simulink model "rx2"  (R2022b)
settings: Solver=FixedStepDiscrete  StartTime=0.0  StopTime=3.3E6  FixedStep=1  RelTol=1e-3  EnableMultiTasking=on
model workspace (MAT data in the model file):
  mwTaskManagerKernelLatency = 0
undefined symbols (not defined in the file or in its folder): Add, jsin, magnitude, rom_pilot_conj_tt, Shift
libraries: hdlsllib x3231, whdlutilities x525, simulink x260, whdlmod x112, whdledac x26, dsphdlmathfun2 x24, commchan3 x1
(part 17 of 59)

== system rx2/process divide/transport_block1/Subsystem2/ctrl_gen ==
  data_in : Inport
  valid_in : Inport  Port=2
  Delay : Delay  DelayLength=1  InitialCondition=0
  Delay1 : Delay  DelayLength=1  InitialCondition=0
  Delay2 : Delay  DelayLength=1  InitialCondition=0
  Detect Fall Nonpositive : hdlsllib/Logic and Bit Operations/Detect Fall Nonpositive  vinit=0  OutDataTypeStr=boolean
  Detect Rise Positive : hdlsllib/Logic and Bit Operations/Detect Rise Positive  vinit=0  OutDataTypeStr=boolean
  Sample Control Bus Creator : whdlutilities/Sample Control Bus Creator
  data_out : Outport
  ctrl_out : Outport  Port=2
  wires:
  Detect Rise Positive/1 -> Sample Control Bus Creator/1
  Delay2/1 -> data_out/1
  data_in/1 -> Delay2/1
  Delay1/1 -> Detect Rise Positive/1
  Delay/1 -> Sample Control Bus Creator/3
  Sample Control Bus Creator/1 -> ctrl_out/1
  valid_in/1 -> Delay1/1, Detect Fall Nonpositive/1, Delay/1
  Detect Fall Nonpositive/1 -> Sample Control Bus Creator/2

== system rx2/process divide/transport_block1/Subsystem3/ctrl_gen ==
  data_in : Inport
  valid_in : Inport  Port=2
  Delay : Delay  DelayLength=1  InitialCondition=0
  Delay1 : Delay  DelayLength=1  InitialCondition=0
  Delay2 : Delay  DelayLength=1  InitialCondition=0
  Detect Fall Nonpositive : hdlsllib/Logic and Bit Operations/Detect Fall Nonpositive  vinit=0  OutDataTypeStr=boolean
  Detect Rise Positive : hdlsllib/Logic and Bit Operations/Detect Rise Positive  vinit=0  OutDataTypeStr=boolean
  Sample Control Bus Creator : whdlutilities/Sample Control Bus Creator
  data_out : Outport
  ctrl_out : Outport  Port=2
  wires:
  Detect Fall Nonpositive/1 -> Sample Control Bus Creator/2
  valid_in/1 -> Delay/1, Detect Fall Nonpositive/1, Delay1/1
  Sample Control Bus Creator/1 -> ctrl_out/1
  Delay/1 -> Sample Control Bus Creator/3
  Delay1/1 -> Detect Rise Positive/1
  data_in/1 -> Delay2/1
  Delay2/1 -> data_out/1
  Detect Rise Positive/1 -> Sample Control Bus Creator/1

== system rx2/process divide/transport_block1/Subsystem4/ctrl_gen ==
  data_in : Inport
  valid_in : Inport  Port=2
  Delay : Delay  DelayLength=1  InitialCondition=0
  Delay1 : Delay  DelayLength=1  InitialCondition=0
  Delay2 : Delay  DelayLength=1  InitialCondition=0
  Detect Fall Nonpositive : hdlsllib/Logic and Bit Operations/Detect Fall Nonpositive  vinit=0  OutDataTypeStr=boolean
  Detect Rise Positive : hdlsllib/Logic and Bit Operations/Detect Rise Positive  vinit=0  OutDataTypeStr=boolean
  Sample Control Bus Creator : whdlutilities/Sample Control Bus Creator
  data_out : Outport
  ctrl_out : Outport  Port=2
  wires:
  Detect Rise Positive/1 -> Sample Control Bus Creator/1
  Delay2/1 -> data_out/1
  data_in/1 -> Delay2/1
  Delay1/1 -> Detect Rise Positive/1
  Delay/1 -> Sample Control Bus Creator/3
  Sample Control Bus Creator/1 -> ctrl_out/1
  valid_in/1 -> Delay1/1, Detect Fall Nonpositive/1, Delay/1
  Detect Fall Nonpositive/1 -> Sample Control Bus Creator/2

== system rx2/process divide/transport_block1/Subsystem5/ctrl_gen ==
  data_in : Inport
  valid_in : Inport  Port=2
  Delay : Delay  DelayLength=1  InitialCondition=0
  Delay1 : Delay  DelayLength=1  InitialCondition=0
  Delay2 : Delay  DelayLength=1  InitialCondition=0
  Detect Fall Nonpositive : hdlsllib/Logic and Bit Operations/Detect Fall Nonpositive  vinit=0  OutDataTypeStr=boolean
  Detect Rise Positive : hdlsllib/Logic and Bit Operations/Detect Rise Positive  vinit=0  OutDataTypeStr=boolean
  Sample Control Bus Creator : whdlutilities/Sample Control Bus Creator
  data_out : Outport
  ctrl_out : Outport  Port=2
  wires:
  Detect Rise Positive/1 -> Sample Control Bus Creator/1
  Delay2/1 -> data_out/1
  data_in/1 -> Delay2/1
  Delay1/1 -> Detect Rise Positive/1
  Delay/1 -> Sample Control Bus Creator/3
  Sample Control Bus Creator/1 -> ctrl_out/1
  valid_in/1 -> Delay1/1, Detect Fall Nonpositive/1, Delay/1
  Detect Fall Nonpositive/1 -> Sample Control Bus Creator/2

== system rx2/process divide/transport_block1/Subsystem6/ctrl_gen ==
  data_in : Inport
  valid_in : Inport  Port=2
  Delay : Delay  DelayLength=1  InitialCondition=0
  Delay1 : Delay  DelayLength=1  InitialCondition=0
  Delay2 : Delay  DelayLength=1  InitialCondition=0
  Detect Fall Nonpositive : hdlsllib/Logic and Bit Operations/Detect Fall Nonpositive  vinit=0  OutDataTypeStr=boolean
  Detect Rise Positive : hdlsllib/Logic and Bit Operations/Detect Rise Positive  vinit=0  OutDataTypeStr=boolean
  Sample Control Bus Creator : whdlutilities/Sample Control Bus Creator
  data_out : Outport
  ctrl_out : Outport  Port=2
  wires:
  Detect Rise Positive/1 -> Sample Control Bus Creator/1
  Delay2/1 -> data_out/1
  data_in/1 -> Delay2/1
  Delay1/1 -> Detect Rise Positive/1
  Delay/1 -> Sample Control Bus Creator/3
  Sample Control Bus Creator/1 -> ctrl_out/1
  valid_in/1 -> Delay1/1, Detect Fall Nonpositive/1, Delay/1
  Detect Fall Nonpositive/1 -> Sample Control Bus Creator/2

== system rx2/process divide/transport_block1/Subsystem7/ctrl_gen ==
  data_in : Inport
  valid_in : Inport  Port=2
  Delay : Delay  DelayLength=1  InitialCondition=0
  Delay1 : Delay  DelayLength=1  InitialCondition=0
  Delay2 : Delay  DelayLength=1  InitialCondition=0
  Detect Fall Nonpositive : hdlsllib/Logic and Bit Operations/Detect Fall Nonpositive  vinit=0  OutDataTypeStr=boolean
  Detect Rise Positive : hdlsllib/Logic and Bit Operations/Detect Rise Positive  vinit=0  OutDataTypeStr=boolean
  Sample Control Bus Creator : whdlutilities/Sample Control Bus Creator
  data_out : Outport
  ctrl_out : Outport  Port=2
  wires:
  Detect Rise Positive/1 -> Sample Control Bus Creator/1
  Delay2/1 -> data_out/1
  data_in/1 -> Delay2/1
  Delay1/1 -> Detect Rise Positive/1
  Delay/1 -> Sample Control Bus Creator/3
  Sample Control Bus Creator/1 -> ctrl_out/1
  valid_in/1 -> Delay1/1, Detect Fall Nonpositive/1, Delay/1
  Detect Fall Nonpositive/1 -> Sample Control Bus Creator/2

== system rx2/process divide/transport_block1/Subsystem8/ctrl_gen ==
  data_in : Inport
  valid_in : Inport  Port=2
  Delay : Delay  DelayLength=1  InitialCondition=0
  Delay1 : Delay  DelayLength=1  InitialCondition=0
  Delay2 : Delay  DelayLength=1  InitialCondition=0
  Detect Fall Nonpositive : hdlsllib/Logic and Bit Operations/Detect Fall Nonpositive  vinit=0  OutDataTypeStr=boolean
  Detect Rise Positive : hdlsllib/Logic and Bit Operations/Detect Rise Positive  vinit=0  OutDataTypeStr=boolean
  Sample Control Bus Creator : whdlutilities/Sample Control Bus Creator
  data_out : Outport
  ctrl_out : Outport  Port=2
  wires:
  Detect Rise Positive/1 -> Sample Control Bus Creator/1
  Delay2/1 -> data_out/1
  data_in/1 -> Delay2/1
  Delay1/1 -> Detect Rise Positive/1
  Delay/1 -> Sample Control Bus Creator/3
  Sample Control Bus Creator/1 -> ctrl_out/1
  valid_in/1 -> Delay1/1, Detect Fall Nonpositive/1, Delay/1
  Detect Fall Nonpositive/1 -> Sample Control Bus Creator/2

== system rx2/process divide/transport_block1/Subsystem9/ctrl_gen ==
  data_in : Inport
  valid_in : Inport  Port=2
  Delay : Delay  DelayLength=1  InitialCondition=0
  Delay1 : Delay  DelayLength=1  InitialCondition=0
  Delay2 : Delay  DelayLength=1  InitialCondition=0
  Detect Fall Nonpositive : hdlsllib/Logic and Bit Operations/Detect Fall Nonpositive  vinit=0  OutDataTypeStr=boolean
  Detect Rise Positive : hdlsllib/Logic and Bit Operations/Detect Rise Positive  vinit=0  OutDataTypeStr=boolean
  Sample Control Bus Creator : whdlutilities/Sample Control Bus Creator
  data_out : Outport
  ctrl_out : Outport  Port=2
  wires:
  Detect Rise Positive/1 -> Sample Control Bus Creator/1
  Delay2/1 -> data_out/1
  data_in/1 -> Delay2/1
  Delay1/1 -> Detect Rise Positive/1
  Delay/1 -> Sample Control Bus Creator/3
  Sample Control Bus Creator/1 -> ctrl_out/1
  valid_in/1 -> Delay1/1, Detect Fall Nonpositive/1, Delay/1
  Detect Fall Nonpositive/1 -> Sample Control Bus Creator/2

== system rx2/process divide/transport_block2/Subsystem1/ctrl_gen ==
  data_in : Inport
  valid_in : Inport  Port=2
  Delay : Delay  DelayLength=1  InitialCondition=0
  Delay1 : Delay  DelayLength=1  InitialCondition=0
  Delay2 : Delay  DelayLength=1  InitialCondition=0
  Detect Fall Nonpositive : hdlsllib/Logic and Bit Operations/Detect Fall Nonpositive  vinit=0  OutDataTypeStr=boolean
  Detect Rise Positive : hdlsllib/Logic and Bit Operations/Detect Rise Positive  vinit=0  OutDataTypeStr=boolean
  Sample Control Bus Creator : whdlutilities/Sample Control Bus Creator
  data_out : Outport
  ctrl_out : Outport  Port=2
  wires:
  Detect Rise Positive/1 -> Sample Control Bus Creator/1
  Delay2/1 -> data_out/1
  data_in/1 -> Delay2/1
  Delay1/1 -> Detect Rise Positive/1
  Delay/1 -> Sample Control Bus Creator/3
  Sample Control Bus Creator/1 -> ctrl_out/1
  valid_in/1 -> Delay1/1, Detect Fall Nonpositive/1, Delay/1
  Detect Fall Nonpositive/1 -> Sample Control Bus Creator/2

== system rx2/process divide/transport_block2/Subsystem10/ctrl_gen ==
  data_in : Inport
  valid_in : Inport  Port=2
  Delay : Delay  DelayLength=1  InitialCondition=0
  Delay1 : Delay  DelayLength=1  InitialCondition=0
  Delay2 : Delay  DelayLength=1  InitialCondition=0
  Detect Fall Nonpositive : hdlsllib/Logic and Bit Operations/Detect Fall Nonpositive  vinit=0  OutDataTypeStr=boolean
  Detect Rise Positive : hdlsllib/Logic and Bit Operations/Detect Rise Positive  vinit=0  OutDataTypeStr=boolean
  Sample Control Bus Creator : whdlutilities/Sample Control Bus Creator
  data_out : Outport
  ctrl_out : Outport  Port=2
  wires:
  Detect Fall Nonpositive/1 -> Sample Control Bus Creator/2
  valid_in/1 -> Delay/1, Detect Fall Nonpositive/1, Delay1/1
  Sample Control Bus Creator/1 -> ctrl_out/1
  Delay/1 -> Sample Control Bus Creator/3
  Delay1/1 -> Detect Rise Positive/1
  data_in/1 -> Delay2/1
  Delay2/1 -> data_out/1
  Detect Rise Positive/1 -> Sample Control Bus Creator/1

== system rx2/process divide/transport_block2/Subsystem11/ctrl_gen ==
  data_in : Inport
  valid_in : Inport  Port=2
  Delay : Delay  DelayLength=1  InitialCondition=0
  Delay1 : Delay  DelayLength=1  InitialCondition=0
  Delay2 : Delay  DelayLength=1  InitialCondition=0
  Detect Fall Nonpositive : hdlsllib/Logic and Bit Operations/Detect Fall Nonpositive  vinit=0  OutDataTypeStr=boolean
  Detect Rise Positive : hdlsllib/Logic and Bit Operations/Detect Rise Positive  vinit=0  OutDataTypeStr=boolean
  Sample Control Bus Creator : whdlutilities/Sample Control Bus Creator
  data_out : Outport
  ctrl_out : Outport  Port=2
  wires:
  Detect Fall Nonpositive/1 -> Sample Control Bus Creator/2
  valid_in/1 -> Delay/1, Detect Fall Nonpositive/1, Delay1/1
  Sample Control Bus Creator/1 -> ctrl_out/1
  Delay/1 -> Sample Control Bus Creator/3
  Delay1/1 -> Detect Rise Positive/1
  data_in/1 -> Delay2/1
  Delay2/1 -> data_out/1
  Detect Rise Positive/1 -> Sample Control Bus Creator/1

== system rx2/process divide/transport_block2/Subsystem12/ctrl_gen ==
  data_in : Inport
  valid_in : Inport  Port=2
  Delay : Delay  DelayLength=1  InitialCondition=0
  Delay1 : Delay  DelayLength=1  InitialCondition=0
  Delay2 : Delay  DelayLength=1  InitialCondition=0
  Detect Fall Nonpositive : hdlsllib/Logic and Bit Operations/Detect Fall Nonpositive  vinit=0  OutDataTypeStr=boolean
  Detect Rise Positive : hdlsllib/Logic and Bit Operations/Detect Rise Positive  vinit=0  OutDataTypeStr=boolean
  Sample Control Bus Creator : whdlutilities/Sample Control Bus Creator
  data_out : Outport
  ctrl_out : Outport  Port=2
  wires:
  Detect Fall Nonpositive/1 -> Sample Control Bus Creator/2
  valid_in/1 -> Delay/1, Detect Fall Nonpositive/1, Delay1/1
  Sample Control Bus Creator/1 -> ctrl_out/1
  Delay/1 -> Sample Control Bus Creator/3
  Delay1/1 -> Detect Rise Positive/1
  data_in/1 -> Delay2/1
  Delay2/1 -> data_out/1
  Detect Rise Positive/1 -> Sample Control Bus Creator/1

== system rx2/process divide/transport_block2/Subsystem13/ctrl_gen ==
  data_in : Inport
  valid_in : Inport  Port=2
  Delay : Delay  DelayLength=1  InitialCondition=0
  Delay1 : Delay  DelayLength=1  InitialCondition=0
  Delay2 : Delay  DelayLength=1  InitialCondition=0
  Detect Fall Nonpositive : hdlsllib/Logic and Bit Operations/Detect Fall Nonpositive  vinit=0  OutDataTypeStr=boolean
  Detect Rise Positive : hdlsllib/Logic and Bit Operations/Detect Rise Positive  vinit=0  OutDataTypeStr=boolean
  Sample Control Bus Creator : whdlutilities/Sample Control Bus Creator
  data_out : Outport
  ctrl_out : Outport  Port=2
  wires:
  Detect Fall Nonpositive/1 -> Sample Control Bus Creator/2
  valid_in/1 -> Delay/1, Detect Fall Nonpositive/1, Delay1/1
  Sample Control Bus Creator/1 -> ctrl_out/1
  Delay/1 -> Sample Control Bus Creator/3
  Delay1/1 -> Detect Rise Positive/1
  data_in/1 -> Delay2/1
  Delay2/1 -> data_out/1
  Detect Rise Positive/1 -> Sample Control Bus Creator/1

== system rx2/process divide/transport_block2/Subsystem14/ctrl_gen ==
  data_in : Inport
  valid_in : Inport  Port=2
  Delay : Delay  DelayLength=1  InitialCondition=0
  Delay1 : Delay  DelayLength=1  InitialCondition=0
  Delay2 : Delay  DelayLength=1  InitialCondition=0
  Detect Fall Nonpositive : hdlsllib/Logic and Bit Operations/Detect Fall Nonpositive  vinit=0  OutDataTypeStr=boolean
  Detect Rise Positive : hdlsllib/Logic and Bit Operations/Detect Rise Positive  vinit=0  OutDataTypeStr=boolean
  Sample Control Bus Creator : whdlutilities/Sample Control Bus Creator
  data_out : Outport
  ctrl_out : Outport  Port=2
  wires:
  Detect Fall Nonpositive/1 -> Sample Control Bus Creator/2
  valid_in/1 -> Delay/1, Detect Fall Nonpositive/1, Delay1/1
  Sample Control Bus Creator/1 -> ctrl_out/1
  Delay/1 -> Sample Control Bus Creator/3
  Delay1/1 -> Detect Rise Positive/1
  data_in/1 -> Delay2/1
  Delay2/1 -> data_out/1
  Detect Rise Positive/1 -> Sample Control Bus Creator/1

== system rx2/process divide/transport_block2/Subsystem2/ctrl_gen ==
  data_in : Inport
  valid_in : Inport  Port=2
  Delay : Delay  DelayLength=1  InitialCondition=0
  Delay1 : Delay  DelayLength=1  InitialCondition=0
  Delay2 : Delay  DelayLength=1  InitialCondition=0
  Detect Fall Nonpositive : hdlsllib/Logic and Bit Operations/Detect Fall Nonpositive  vinit=0  OutDataTypeStr=boolean
  Detect Rise Positive : hdlsllib/Logic and Bit Operations/Detect Rise Positive  vinit=0  OutDataTypeStr=boolean
  Sample Control Bus Creator : whdlutilities/Sample Control Bus Creator
  data_out : Outport
  ctrl_out : Outport  Port=2
  wires:
  Detect Fall Nonpositive/1 -> Sample Control Bus Creator/2
  valid_in/1 -> Delay/1, Detect Fall Nonpositive/1, Delay1/1
  Sample Control Bus Creator/1 -> ctrl_out/1
  Delay/1 -> Sample Control Bus Creator/3
  Delay1/1 -> Detect Rise Positive/1
  data_in/1 -> Delay2/1
  Delay2/1 -> data_out/1
  Detect Rise Positive/1 -> Sample Control Bus Creator/1

== system rx2/process divide/transport_block2/Subsystem3/ctrl_gen ==
  data_in : Inport
  valid_in : Inport  Port=2
  Delay : Delay  DelayLength=1  InitialCondition=0
  Delay1 : Delay  DelayLength=1  InitialCondition=0
  Delay2 : Delay  DelayLength=1  InitialCondition=0
  Detect Fall Nonpositive : hdlsllib/Logic and Bit Operations/Detect Fall Nonpositive  vinit=0  OutDataTypeStr=boolean
  Detect Rise Positive : hdlsllib/Logic and Bit Operations/Detect Rise Positive  vinit=0  OutDataTypeStr=boolean
  Sample Control Bus Creator : whdlutilities/Sample Control Bus Creator
  data_out : Outport
  ctrl_out : Outport  Port=2
  wires:
  Detect Rise Positive/1 -> Sample Control Bus Creator/1
  Delay2/1 -> data_out/1
  data_in/1 -> Delay2/1
  Delay1/1 -> Detect Rise Positive/1
  Delay/1 -> Sample Control Bus Creator/3
  Sample Control Bus Creator/1 -> ctrl_out/1
  valid_in/1 -> Delay1/1, Detect Fall Nonpositive/1, Delay/1
  Detect Fall Nonpositive/1 -> Sample Control Bus Creator/2

== system rx2/process divide/transport_block2/Subsystem4/ctrl_gen ==
  data_in : Inport
  valid_in : Inport  Port=2
  Delay : Delay  DelayLength=1  InitialCondition=0
  Delay1 : Delay  DelayLength=1  InitialCondition=0
  Delay2 : Delay  DelayLength=1  InitialCondition=0
  Detect Fall Nonpositive : hdlsllib/Logic and Bit Operations/Detect Fall Nonpositive  vinit=0  OutDataTypeStr=boolean
  Detect Rise Positive : hdlsllib/Logic and Bit Operations/Detect Rise Positive  vinit=0  OutDataTypeStr=boolean
  Sample Control Bus Creator : whdlutilities/Sample Control Bus Creator
  data_out : Outport
  ctrl_out : Outport  Port=2
  wires:
  Detect Fall Nonpositive/1 -> Sample Control Bus Creator/2
  valid_in/1 -> Delay/1, Detect Fall Nonpositive/1, Delay1/1
  Sample Control Bus Creator/1 -> ctrl_out/1
  Delay/1 -> Sample Control Bus Creator/3
  Delay1/1 -> Detect Rise Positive/1
  data_in/1 -> Delay2/1
  Delay2/1 -> data_out/1
  Detect Rise Positive/1 -> Sample Control Bus Creator/1

== system rx2/process divide/transport_block2/Subsystem5/ctrl_gen ==
  data_in : Inport
  valid_in : Inport  Port=2
  Delay : Delay  DelayLength=1  InitialCondition=0
  Delay1 : Delay  DelayLength=1  InitialCondition=0
  Delay2 : Delay  DelayLength=1  InitialCondition=0
  Detect Fall Nonpositive : hdlsllib/Logic and Bit Operations/Detect Fall Nonpositive  vinit=0  OutDataTypeStr=boolean
  Detect Rise Positive : hdlsllib/Logic and Bit Operations/Detect Rise Positive  vinit=0  OutDataTypeStr=boolean
  Sample Control Bus Creator : whdlutilities/Sample Control Bus Creator
  data_out : Outport
  ctrl_out : Outport  Port=2
  wires:
  Detect Fall Nonpositive/1 -> Sample Control Bus Creator/2
  valid_in/1 -> Delay/1, Detect Fall Nonpositive/1, Delay1/1
  Sample Control Bus Creator/1 -> ctrl_out/1
  Delay/1 -> Sample Control Bus Creator/3
  Delay1/1 -> Detect Rise Positive/1
  data_in/1 -> Delay2/1
  Delay2/1 -> data_out/1
  Detect Rise Positive/1 -> Sample Control Bus Creator/1

== system rx2/process divide/transport_block2/Subsystem6/ctrl_gen ==
  data_in : Inport
  valid_in : Inport  Port=2
  Delay : Delay  DelayLength=1  InitialCondition=0
  Delay1 : Delay  DelayLength=1  InitialCondition=0
  Delay2 : Delay  DelayLength=1  InitialCondition=0
  Detect Fall Nonpositive : hdlsllib/Logic and Bit Operations/Detect Fall Nonpositive  vinit=0  OutDataTypeStr=boolean
  Detect Rise Positive : hdlsllib/Logic and Bit Operations/Detect Rise Positive  vinit=0  OutDataTypeStr=boolean
  Sample Control Bus Creator : whdlutilities/Sample Control Bus Creator
  data_out : Outport
  ctrl_out : Outport  Port=2
  wires:
  Detect Fall Nonpositive/1 -> Sample Control Bus Creator/2
  valid_in/1 -> Delay/1, Detect Fall Nonpositive/1, Delay1/1
  Sample Control Bus Creator/1 -> ctrl_out/1
  Delay/1 -> Sample Control Bus Creator/3
  Delay1/1 -> Detect Rise Positive/1
  data_in/1 -> Delay2/1
  Delay2/1 -> data_out/1
  Detect Rise Positive/1 -> Sample Control Bus Creator/1

== system rx2/process divide/transport_block2/Subsystem7/ctrl_gen ==
  data_in : Inport
  valid_in : Inport  Port=2
  Delay : Delay  DelayLength=1  InitialCondition=0
  Delay1 : Delay  DelayLength=1  InitialCondition=0
  Delay2 : Delay  DelayLength=1  InitialCondition=0
  Detect Fall Nonpositive : hdlsllib/Logic and Bit Operations/Detect Fall Nonpositive  vinit=0  OutDataTypeStr=boolean
  Detect Rise Positive : hdlsllib/Logic and Bit Operations/Detect Rise Positive  vinit=0  OutDataTypeStr=boolean
  Sample Control Bus Creator : whdlutilities/Sample Control Bus Creator
  data_out : Outport
  ctrl_out : Outport  Port=2
  wires:
  Detect Fall Nonpositive/1 -> Sample Control Bus Creator/2
  valid_in/1 -> Delay/1, Detect Fall Nonpositive/1, Delay1/1
  Sample Control Bus Creator/1 -> ctrl_out/1
  Delay/1 -> Sample Control Bus Creator/3
  Delay1/1 -> Detect Rise Positive/1
  data_in/1 -> Delay2/1
  Delay2/1 -> data_out/1
  Detect Rise Positive/1 -> Sample Control Bus Creator/1

== system rx2/process divide/transport_block2/Subsystem8/ctrl_gen ==
  data_in : Inport
  valid_in : Inport  Port=2
  Delay : Delay  DelayLength=1  InitialCondition=0
  Delay1 : Delay  DelayLength=1  InitialCondition=0
  Delay2 : Delay  DelayLength=1  InitialCondition=0
  Detect Fall Nonpositive : hdlsllib/Logic and Bit Operations/Detect Fall Nonpositive  vinit=0  OutDataTypeStr=boolean
  Detect Rise Positive : hdlsllib/Logic and Bit Operations/Detect Rise Positive  vinit=0  OutDataTypeStr=boolean
  Sample Control Bus Creator : whdlutilities/Sample Control Bus Creator
  data_out : Outport
  ctrl_out : Outport  Port=2
  wires:
  Detect Fall Nonpositive/1 -> Sample Control Bus Creator/2
  valid_in/1 -> Delay/1, Detect Fall Nonpositive/1, Delay1/1
  Sample Control Bus Creator/1 -> ctrl_out/1
  Delay/1 -> Sample Control Bus Creator/3
  Delay1/1 -> Detect Rise Positive/1
  data_in/1 -> Delay2/1
  Delay2/1 -> data_out/1
  Detect Rise Positive/1 -> Sample Control Bus Creator/1

== system rx2/process divide/transport_block2/Subsystem9/ctrl_gen ==
  data_in : Inport
  valid_in : Inport  Port=2
  Delay : Delay  DelayLength=1  InitialCondition=0
  Delay1 : Delay  DelayLength=1  InitialCondition=0
  Delay2 : Delay  DelayLength=1  InitialCondition=0
  Detect Fall Nonpositive : hdlsllib/Logic and Bit Operations/Detect Fall Nonpositive  vinit=0  OutDataTypeStr=boolean
  Detect Rise Positive : hdlsllib/Logic and Bit Operations/Detect Rise Positive  vinit=0  OutDataTypeStr=boolean
  Sample Control Bus Creator : whdlutilities/Sample Control Bus Creator
  data_out : Outport
  ctrl_out : Outport  Port=2
  wires:
  Detect Fall Nonpositive/1 -> Sample Control Bus Creator/2
  valid_in/1 -> Delay/1, Detect Fall Nonpositive/1, Delay1/1
  Sample Control Bus Creator/1 -> ctrl_out/1
  Delay/1 -> Sample Control Bus Creator/3
  Delay1/1 -> Detect Rise Positive/1
  data_in/1 -> Delay2/1
  Delay2/1 -> data_out/1
  Detect Rise Positive/1 -> Sample Control Bus Creator/1

== system rx2/process divide/transport_block3/Subsystem1/ctrl_gen ==
  data_in : Inport
  valid_in : Inport  Port=2
  Delay : Delay  DelayLength=1  InitialCondition=0
  Delay1 : Delay  DelayLength=1  InitialCondition=0
  Delay2 : Delay  DelayLength=1  InitialCondition=0
  Detect Fall Nonpositive : hdlsllib/Logic and Bit Operations/Detect Fall Nonpositive  vinit=0  OutDataTypeStr=boolean
  Detect Rise Positive : hdlsllib/Logic and Bit Operations/Detect Rise Positive  vinit=0  OutDataTypeStr=boolean
  Sample Control Bus Creator : whdlutilities/Sample Control Bus Creator
  data_out : Outport
  ctrl_out : Outport  Port=2
  wires:
  Detect Fall Nonpositive/1 -> Sample Control Bus Creator/2
  valid_in/1 -> Delay/1, Detect Fall Nonpositive/1, Delay1/1
  Sample Control Bus Creator/1 -> ctrl_out/1
  Delay/1 -> Sample Control Bus Creator/3
  Delay1/1 -> Detect Rise Positive/1
  data_in/1 -> Delay2/1
  Delay2/1 -> data_out/1
  Detect Rise Positive/1 -> Sample Control Bus Creator/1

== system rx2/process divide/transport_block3/Subsystem10/ctrl_gen ==
  data_in : Inport
  valid_in : Inport  Port=2
  Delay : Delay  DelayLength=1  InitialCondition=0
  Delay1 : Delay  DelayLength=1  InitialCondition=0
  Delay2 : Delay  DelayLength=1  InitialCondition=0
  Detect Fall Nonpositive : hdlsllib/Logic and Bit Operations/Detect Fall Nonpositive  vinit=0  OutDataTypeStr=boolean
  Detect Rise Positive : hdlsllib/Logic and Bit Operations/Detect Rise Positive  vinit=0  OutDataTypeStr=boolean
  Sample Control Bus Creator : whdlutilities/Sample Control Bus Creator
  data_out : Outport
  ctrl_out : Outport  Port=2
  wires:
  Detect Rise Positive/1 -> Sample Control Bus Creator/1
  Delay2/1 -> data_out/1
  data_in/1 -> Delay2/1
  Delay1/1 -> Detect Rise Positive/1
  Delay/1 -> Sample Control Bus Creator/3
  Sample Control Bus Creator/1 -> ctrl_out/1
  valid_in/1 -> Delay1/1, Detect Fall Nonpositive/1, Delay/1
  Detect Fall Nonpositive/1 -> Sample Control Bus Creator/2

== system rx2/process divide/transport_block3/Subsystem11/ctrl_gen ==
  data_in : Inport
  valid_in : Inport  Port=2
  Delay : Delay  DelayLength=1  InitialCondition=0
  Delay1 : Delay  DelayLength=1  InitialCondition=0
  Delay2 : Delay  DelayLength=1  InitialCondition=0
  Detect Fall Nonpositive : hdlsllib/Logic and Bit Operations/Detect Fall Nonpositive  vinit=0  OutDataTypeStr=boolean
  Detect Rise Positive : hdlsllib/Logic and Bit Operations/Detect Rise Positive  vinit=0  OutDataTypeStr=boolean
  Sample Control Bus Creator : whdlutilities/Sample Control Bus Creator
  data_out : Outport
  ctrl_out : Outport  Port=2
  wires:
  Detect Rise Positive/1 -> Sample Control Bus Creator/1
  Delay2/1 -> data_out/1
  data_in/1 -> Delay2/1
  Delay1/1 -> Detect Rise Positive/1
  Delay/1 -> Sample Control Bus Creator/3
  Sample Control Bus Creator/1 -> ctrl_out/1
  valid_in/1 -> Delay1/1, Detect Fall Nonpositive/1, Delay/1
  Detect Fall Nonpositive/1 -> Sample Control Bus Creator/2

== system rx2/process divide/transport_block3/Subsystem12/ctrl_gen ==
  data_in : Inport
  valid_in : Inport  Port=2
  Delay : Delay  DelayLength=1  InitialCondition=0
  Delay1 : Delay  DelayLength=1  InitialCondition=0
  Delay2 : Delay  DelayLength=1  InitialCondition=0
  Detect Fall Nonpositive : hdlsllib/Logic and Bit Operations/Detect Fall Nonpositive  vinit=0  OutDataTypeStr=boolean
  Detect Rise Positive : hdlsllib/Logic and Bit Operations/Detect Rise Positive  vinit=0  OutDataTypeStr=boolean
  Sample Control Bus Creator : whdlutilities/Sample Control Bus Creator
  data_out : Outport
  ctrl_out : Outport  Port=2
  wires:
  Detect Rise Positive/1 -> Sample Control Bus Creator/1
  Delay2/1 -> data_out/1
  data_in/1 -> Delay2/1
  Delay1/1 -> Detect Rise Positive/1
  Delay/1 -> Sample Control Bus Creator/3
  Sample Control Bus Creator/1 -> ctrl_out/1
  valid_in/1 -> Delay1/1, Detect Fall Nonpositive/1, Delay/1
  Detect Fall Nonpositive/1 -> Sample Control Bus Creator/2

== system rx2/process divide/transport_block3/Subsystem13/ctrl_gen ==
  data_in : Inport
  valid_in : Inport  Port=2
  Delay : Delay  DelayLength=1  InitialCondition=0
  Delay1 : Delay  DelayLength=1  InitialCondition=0
  Delay2 : Delay  DelayLength=1  InitialCondition=0
  Detect Fall Nonpositive : hdlsllib/Logic and Bit Operations/Detect Fall Nonpositive  vinit=0  OutDataTypeStr=boolean
  Detect Rise Positive : hdlsllib/Logic and Bit Operations/Detect Rise Positive  vinit=0  OutDataTypeStr=boolean
  Sample Control Bus Creator : whdlutilities/Sample Control Bus Creator
  data_out : Outport
  ctrl_out : Outport  Port=2
  wires:
  Detect Rise Positive/1 -> Sample Control Bus Creator/1
  Delay2/1 -> data_out/1
  data_in/1 -> Delay2/1
  Delay1/1 -> Detect Rise Positive/1
  Delay/1 -> Sample Control Bus Creator/3
  Sample Control Bus Creator/1 -> ctrl_out/1
  valid_in/1 -> Delay1/1, Detect Fall Nonpositive/1, Delay/1
  Detect Fall Nonpositive/1 -> Sample Control Bus Creator/2

== system rx2/process divide/transport_block3/Subsystem14/ctrl_gen ==
  data_in : Inport
  valid_in : Inport  Port=2
  Delay : Delay  DelayLength=1  InitialCondition=0
  Delay1 : Delay  DelayLength=1  InitialCondition=0
  Delay2 : Delay  DelayLength=1  InitialCondition=0
  Detect Fall Nonpositive : hdlsllib/Logic and Bit Operations/Detect Fall Nonpositive  vinit=0  OutDataTypeStr=boolean
  Detect Rise Positive : hdlsllib/Logic and Bit Operations/Detect Rise Positive  vinit=0  OutDataTypeStr=boolean
  Sample Control Bus Creator : whdlutilities/Sample Control Bus Creator
  data_out : Outport
  ctrl_out : Outport  Port=2
  wires:
  Detect Rise Positive/1 -> Sample Control Bus Creator/1
  Delay2/1 -> data_out/1
  data_in/1 -> Delay2/1
  Delay1/1 -> Detect Rise Positive/1
  Delay/1 -> Sample Control Bus Creator/3
  Sample Control Bus Creator/1 -> ctrl_out/1
  valid_in/1 -> Delay1/1, Detect Fall Nonpositive/1, Delay/1
  Detect Fall Nonpositive/1 -> Sample Control Bus Creator/2

== system rx2/process divide/transport_block3/Subsystem2/ctrl_gen ==
  data_in : Inport
  valid_in : Inport  Port=2
  Delay : Delay  DelayLength=1  InitialCondition=0
  Delay1 : Delay  DelayLength=1  InitialCondition=0
  Delay2 : Delay  DelayLength=1  InitialCondition=0
  Detect Fall Nonpositive : hdlsllib/Logic and Bit Operations/Detect Fall Nonpositive  vinit=0  OutDataTypeStr=boolean
  Detect Rise Positive : hdlsllib/Logic and Bit Operations/Detect Rise Positive  vinit=0  OutDataTypeStr=boolean
  Sample Control Bus Creator : whdlutilities/Sample Control Bus Creator
  data_out : Outport
  ctrl_out : Outport  Port=2
  wires:
  Detect Rise Positive/1 -> Sample Control Bus Creator/1
  Delay2/1 -> data_out/1
  data_in/1 -> Delay2/1
  Delay1/1 -> Detect Rise Positive/1
  Delay/1 -> Sample Control Bus Creator/3
  Sample Control Bus Creator/1 -> ctrl_out/1
  valid_in/1 -> Delay1/1, Detect Fall Nonpositive/1, Delay/1
  Detect Fall Nonpositive/1 -> Sample Control Bus Creator/2

== system rx2/process divide/transport_block3/Subsystem3/ctrl_gen ==
  data_in : Inport
  valid_in : Inport  Port=2
  Delay : Delay  DelayLength=1  InitialCondition=0
  Delay1 : Delay  DelayLength=1  InitialCondition=0
  Delay2 : Delay  DelayLength=1  InitialCondition=0
  Detect Fall Nonpositive : hdlsllib/Logic and Bit Operations/Detect Fall Nonpositive  vinit=0  OutDataTypeStr=boolean
  Detect Rise Positive : hdlsllib/Logic and Bit Operations/Detect Rise Positive  vinit=0  OutDataTypeStr=boolean
  Sample Control Bus Creator : whdlutilities/Sample Control Bus Creator
  data_out : Outport
  ctrl_out : Outport  Port=2
  wires:
  Detect Fall Nonpositive/1 -> Sample Control Bus Creator/2
  valid_in/1 -> Delay/1, Detect Fall Nonpositive/1, Delay1/1
  Sample Control Bus Creator/1 -> ctrl_out/1
  Delay/1 -> Sample Control Bus Creator/3
  Delay1/1 -> Detect Rise Positive/1
  data_in/1 -> Delay2/1
  Delay2/1 -> data_out/1
  Detect Rise Positive/1 -> Sample Control Bus Creator/1

== system rx2/process divide/transport_block3/Subsystem4/ctrl_gen ==
  data_in : Inport
  valid_in : Inport  Port=2
  Delay : Delay  DelayLength=1  InitialCondition=0
  Delay1 : Delay  DelayLength=1  InitialCondition=0
  Delay2 : Delay  DelayLength=1  InitialCondition=0
  Detect Fall Nonpositive : hdlsllib/Logic and Bit Operations/Detect Fall Nonpositive  vinit=0  OutDataTypeStr=boolean
  Detect Rise Positive : hdlsllib/Logic and Bit Operations/Detect Rise Positive  vinit=0  OutDataTypeStr=boolean
  Sample Control Bus Creator : whdlutilities/Sample Control Bus Creator
  data_out : Outport
  ctrl_out : Outport  Port=2
  wires:
  Detect Rise Positive/1 -> Sample Control Bus Creator/1
  Delay2/1 -> data_out/1
  data_in/1 -> Delay2/1
  Delay1/1 -> Detect Rise Positive/1
  Delay/1 -> Sample Control Bus Creator/3
  Sample Control Bus Creator/1 -> ctrl_out/1
  valid_in/1 -> Delay1/1, Detect Fall Nonpositive/1, Delay/1
  Detect Fall Nonpositive/1 -> Sample Control Bus Creator/2

== system rx2/process divide/transport_block3/Subsystem5/ctrl_gen ==
  data_in : Inport
  valid_in : Inport  Port=2
  Delay : Delay  DelayLength=1  InitialCondition=0
  Delay1 : Delay  DelayLength=1  InitialCondition=0
  Delay2 : Delay  DelayLength=1  InitialCondition=0
  Detect Fall Nonpositive : hdlsllib/Logic and Bit Operations/Detect Fall Nonpositive  vinit=0  OutDataTypeStr=boolean
  Detect Rise Positive : hdlsllib/Logic and Bit Operations/Detect Rise Positive  vinit=0  OutDataTypeStr=boolean
  Sample Control Bus Creator : whdlutilities/Sample Control Bus Creator
  data_out : Outport
  ctrl_out : Outport  Port=2
  wires:
  Detect Rise Positive/1 -> Sample Control Bus Creator/1
  Delay2/1 -> data_out/1
  data_in/1 -> Delay2/1
  Delay1/1 -> Detect Rise Positive/1
  Delay/1 -> Sample Control Bus Creator/3
  Sample Control Bus Creator/1 -> ctrl_out/1
  valid_in/1 -> Delay1/1, Detect Fall Nonpositive/1, Delay/1
  Detect Fall Nonpositive/1 -> Sample Control Bus Creator/2

== system rx2/process divide/transport_block3/Subsystem6/ctrl_gen ==
  data_in : Inport
  valid_in : Inport  Port=2
  Delay : Delay  DelayLength=1  InitialCondition=0
  Delay1 : Delay  DelayLength=1  InitialCondition=0
  Delay2 : Delay  DelayLength=1  InitialCondition=0
  Detect Fall Nonpositive : hdlsllib/Logic and Bit Operations/Detect Fall Nonpositive  vinit=0  OutDataTypeStr=boolean
  Detect Rise Positive : hdlsllib/Logic and Bit Operations/Detect Rise Positive  vinit=0  OutDataTypeStr=boolean
  Sample Control Bus Creator : whdlutilities/Sample Control Bus Creator
  data_out : Outport
  ctrl_out : Outport  Port=2
  wires:
  Detect Rise Positive/1 -> Sample Control Bus Creator/1
  Delay2/1 -> data_out/1
  data_in/1 -> Delay2/1
  Delay1/1 -> Detect Rise Positive/1
  Delay/1 -> Sample Control Bus Creator/3
  Sample Control Bus Creator/1 -> ctrl_out/1
  valid_in/1 -> Delay1/1, Detect Fall Nonpositive/1, Delay/1
  Detect Fall Nonpositive/1 -> Sample Control Bus Creator/2

== system rx2/process divide/transport_block3/Subsystem7/ctrl_gen ==
  data_in : Inport
  valid_in : Inport  Port=2
  Delay : Delay  DelayLength=1  InitialCondition=0
  Delay1 : Delay  DelayLength=1  InitialCondition=0
  Delay2 : Delay  DelayLength=1  InitialCondition=0
  Detect Fall Nonpositive : hdlsllib/Logic and Bit Operations/Detect Fall Nonpositive  vinit=0  OutDataTypeStr=boolean
  Detect Rise Positive : hdlsllib/Logic and Bit Operations/Detect Rise Positive  vinit=0  OutDataTypeStr=boolean
  Sample Control Bus Creator : whdlutilities/Sample Control Bus Creator
  data_out : Outport
  ctrl_out : Outport  Port=2
  wires:
  Detect Rise Positive/1 -> Sample Control Bus Creator/1
  Delay2/1 -> data_out/1
  data_in/1 -> Delay2/1
  Delay1/1 -> Detect Rise Positive/1
  Delay/1 -> Sample Control Bus Creator/3
  Sample Control Bus Creator/1 -> ctrl_out/1
  valid_in/1 -> Delay1/1, Detect Fall Nonpositive/1, Delay/1
  Detect Fall Nonpositive/1 -> Sample Control Bus Creator/2

== system rx2/process divide/transport_block3/Subsystem8/ctrl_gen ==
  data_in : Inport
  valid_in : Inport  Port=2
  Delay : Delay  DelayLength=1  InitialCondition=0
  Delay1 : Delay  DelayLength=1  InitialCondition=0
  Delay2 : Delay  DelayLength=1  InitialCondition=0
  Detect Fall Nonpositive : hdlsllib/Logic and Bit Operations/Detect Fall Nonpositive  vinit=0  OutDataTypeStr=boolean
  Detect Rise Positive : hdlsllib/Logic and Bit Operations/Detect Rise Positive  vinit=0  OutDataTypeStr=boolean
  Sample Control Bus Creator : whdlutilities/Sample Control Bus Creator
  data_out : Outport
  ctrl_out : Outport  Port=2
  wires:
  Detect Rise Positive/1 -> Sample Control Bus Creator/1
  Delay2/1 -> data_out/1
  data_in/1 -> Delay2/1
  Delay1/1 -> Detect Rise Positive/1
  Delay/1 -> Sample Control Bus Creator/3
  Sample Control Bus Creator/1 -> ctrl_out/1
  valid_in/1 -> Delay1/1, Detect Fall Nonpositive/1, Delay/1
  Detect Fall Nonpositive/1 -> Sample Control Bus Creator/2

== system rx2/process divide/transport_block3/Subsystem9/ctrl_gen ==
  data_in : Inport
  valid_in : Inport  Port=2
  Delay : Delay  DelayLength=1  InitialCondition=0
  Delay1 : Delay  DelayLength=1  InitialCondition=0
  Delay2 : Delay  DelayLength=1  InitialCondition=0
  Detect Fall Nonpositive : hdlsllib/Logic and Bit Operations/Detect Fall Nonpositive  vinit=0  OutDataTypeStr=boolean
  Detect Rise Positive : hdlsllib/Logic and Bit Operations/Detect Rise Positive  vinit=0  OutDataTypeStr=boolean
  Sample Control Bus Creator : whdlutilities/Sample Control Bus Creator
  data_out : Outport
  ctrl_out : Outport  Port=2
  wires:
  Detect Rise Positive/1 -> Sample Control Bus Creator/1
  Delay2/1 -> data_out/1
  data_in/1 -> Delay2/1
  Delay1/1 -> Detect Rise Positive/1
  Delay/1 -> Sample Control Bus Creator/3
  Sample Control Bus Creator/1 -> ctrl_out/1
  valid_in/1 -> Delay1/1, Detect Fall Nonpositive/1, Delay/1
  Detect Fall Nonpositive/1 -> Sample Control Bus Creator/2

== system rx2/process divide/transport_block4/Subsystem1/ctrl_gen ==
  data_in : Inport
  valid_in : Inport  Port=2
  Delay : Delay  DelayLength=1  InitialCondition=0
  Delay1 : Delay  DelayLength=1  InitialCondition=0
  Delay2 : Delay  DelayLength=1  InitialCondition=0
  Detect Fall Nonpositive : hdlsllib/Logic and Bit Operations/Detect Fall Nonpositive  vinit=0  OutDataTypeStr=boolean
  Detect Rise Positive : hdlsllib/Logic and Bit Operations/Detect Rise Positive  vinit=0  OutDataTypeStr=boolean
  Sample Control Bus Creator : whdlutilities/Sample Control Bus Creator
  data_out : Outport
  ctrl_out : Outport  Port=2
  wires:
  Detect Rise Positive/1 -> Sample Control Bus Creator/1
  Delay2/1 -> data_out/1
  data_in/1 -> Delay2/1
  Delay1/1 -> Detect Rise Positive/1
  Delay/1 -> Sample Control Bus Creator/3
  Sample Control Bus Creator/1 -> ctrl_out/1
  valid_in/1 -> Delay1/1, Detect Fall Nonpositive/1, Delay/1
  Detect Fall Nonpositive/1 -> Sample Control Bus Creator/2

== system rx2/process divide/transport_block4/Subsystem10/ctrl_gen ==
  data_in : Inport
  valid_in : Inport  Port=2
  Delay : Delay  DelayLength=1  InitialCondition=0
  Delay1 : Delay  DelayLength=1  InitialCondition=0
  Delay2 : Delay  DelayLength=1  InitialCondition=0
  Detect Fall Nonpositive : hdlsllib/Logic and Bit Operations/Detect Fall Nonpositive  vinit=0  OutDataTypeStr=boolean
  Detect Rise Positive : hdlsllib/Logic and Bit Operations/Detect Rise Positive  vinit=0  OutDataTypeStr=boolean
  Sample Control Bus Creator : whdlutilities/Sample Control Bus Creator
  data_out : Outport
  ctrl_out : Outport  Port=2
  wires:
  Detect Fall Nonpositive/1 -> Sample Control Bus Creator/2
  valid_in/1 -> Delay/1, Detect Fall Nonpositive/1, Delay1/1
  Sample Control Bus Creator/1 -> ctrl_out/1
  Delay/1 -> Sample Control Bus Creator/3
  Delay1/1 -> Detect Rise Positive/1
  data_in/1 -> Delay2/1
  Delay2/1 -> data_out/1
  Detect Rise Positive/1 -> Sample Control Bus Creator/1

== system rx2/process divide/transport_block4/Subsystem11/ctrl_gen ==
  data_in : Inport
  valid_in : Inport  Port=2
  Delay : Delay  DelayLength=1  InitialCondition=0
  Delay1 : Delay  DelayLength=1  InitialCondition=0
  Delay2 : Delay  DelayLength=1  InitialCondition=0
  Detect Fall Nonpositive : hdlsllib/Logic and Bit Operations/Detect Fall Nonpositive  vinit=0  OutDataTypeStr=boolean
  Detect Rise Positive : hdlsllib/Logic and Bit Operations/Detect Rise Positive  vinit=0  OutDataTypeStr=boolean
  Sample Control Bus Creator : whdlutilities/Sample Control Bus Creator
  data_out : Outport
  ctrl_out : Outport  Port=2
  wires:
  Detect Fall Nonpositive/1 -> Sample Control Bus Creator/2
  valid_in/1 -> Delay/1, Detect Fall Nonpositive/1, Delay1/1
  Sample Control Bus Creator/1 -> ctrl_out/1
  Delay/1 -> Sample Control Bus Creator/3
  Delay1/1 -> Detect Rise Positive/1
  data_in/1 -> Delay2/1
  Delay2/1 -> data_out/1
  Detect Rise Positive/1 -> Sample Control Bus Creator/1

== system rx2/process divide/transport_block4/Subsystem12/ctrl_gen ==
  data_in : Inport
  valid_in : Inport  Port=2
  Delay : Delay  DelayLength=1  InitialCondition=0
  Delay1 : Delay  DelayLength=1  InitialCondition=0
  Delay2 : Delay  DelayLength=1  InitialCondition=0
  Detect Fall Nonpositive : hdlsllib/Logic and Bit Operations/Detect Fall Nonpositive  vinit=0  OutDataTypeStr=boolean
  Detect Rise Positive : hdlsllib/Logic and Bit Operations/Detect Rise Positive  vinit=0  OutDataTypeStr=boolean
  Sample Control Bus Creator : whdlutilities/Sample Control Bus Creator
  data_out : Outport
  ctrl_out : Outport  Port=2
  wires:
  Detect Fall Nonpositive/1 -> Sample Control Bus Creator/2
  valid_in/1 -> Delay/1, Detect Fall Nonpositive/1, Delay1/1
  Sample Control Bus Creator/1 -> ctrl_out/1
  Delay/1 -> Sample Control Bus Creator/3
  Delay1/1 -> Detect Rise Positive/1
  data_in/1 -> Delay2/1
  Delay2/1 -> data_out/1
  Detect Rise Positive/1 -> Sample Control Bus Creator/1

== system rx2/process divide/transport_block4/Subsystem13/ctrl_gen ==
  data_in : Inport
  valid_in : Inport  Port=2
  Delay : Delay  DelayLength=1  InitialCondition=0
  Delay1 : Delay  DelayLength=1  InitialCondition=0
  Delay2 : Delay  DelayLength=1  InitialCondition=0
  Detect Fall Nonpositive : hdlsllib/Logic and Bit Operations/Detect Fall Nonpositive  vinit=0  OutDataTypeStr=boolean
  Detect Rise Positive : hdlsllib/Logic and Bit Operations/Detect Rise Positive  vinit=0  OutDataTypeStr=boolean
  Sample Control Bus Creator : whdlutilities/Sample Control Bus Creator
  data_out : Outport
  ctrl_out : Outport  Port=2
  wires:
  Detect Fall Nonpositive/1 -> Sample Control Bus Creator/2
  valid_in/1 -> Delay/1, Detect Fall Nonpositive/1, Delay1/1
  Sample Control Bus Creator/1 -> ctrl_out/1
  Delay/1 -> Sample Control Bus Creator/3
  Delay1/1 -> Detect Rise Positive/1
  data_in/1 -> Delay2/1
  Delay2/1 -> data_out/1
  Detect Rise Positive/1 -> Sample Control Bus Creator/1

== system rx2/process divide/transport_block4/Subsystem14/ctrl_gen ==
  data_in : Inport
  valid_in : Inport  Port=2
  Delay : Delay  DelayLength=1  InitialCondition=0
  Delay1 : Delay  DelayLength=1  InitialCondition=0
  Delay2 : Delay  DelayLength=1  InitialCondition=0
  Detect Fall Nonpositive : hdlsllib/Logic and Bit Operations/Detect Fall Nonpositive  vinit=0  OutDataTypeStr=boolean
  Detect Rise Positive : hdlsllib/Logic and Bit Operations/Detect Rise Positive  vinit=0  OutDataTypeStr=boolean
  Sample Control Bus Creator : whdlutilities/Sample Control Bus Creator
  data_out : Outport
  ctrl_out : Outport  Port=2
  wires:
  Detect Fall Nonpositive/1 -> Sample Control Bus Creator/2
  valid_in/1 -> Delay/1, Detect Fall Nonpositive/1, Delay1/1
  Sample Control Bus Creator/1 -> ctrl_out/1
  Delay/1 -> Sample Control Bus Creator/3
  Delay1/1 -> Detect Rise Positive/1
  data_in/1 -> Delay2/1
  Delay2/1 -> data_out/1
  Detect Rise Positive/1 -> Sample Control Bus Creator/1

== system rx2/process divide/transport_block4/Subsystem2/ctrl_gen ==
  data_in : Inport
  valid_in : Inport  Port=2
  Delay : Delay  DelayLength=1  InitialCondition=0
  Delay1 : Delay  DelayLength=1  InitialCondition=0
  Delay2 : Delay  DelayLength=1  InitialCondition=0
  Detect Fall Nonpositive : hdlsllib/Logic and Bit Operations/Detect Fall Nonpositive  vinit=0  OutDataTypeStr=boolean
  Detect Rise Positive : hdlsllib/Logic and Bit Operations/Detect Rise Positive  vinit=0  OutDataTypeStr=boolean
  Sample Control Bus Creator : whdlutilities/Sample Control Bus Creator
  data_out : Outport
  ctrl_out : Outport  Port=2
  wires:
  Detect Fall Nonpositive/1 -> Sample Control Bus Creator/2
  valid_in/1 -> Delay/1, Detect Fall Nonpositive/1, Delay1/1
  Sample Control Bus Creator/1 -> ctrl_out/1
  Delay/1 -> Sample Control Bus Creator/3
  Delay1/1 -> Detect Rise Positive/1
  data_in/1 -> Delay2/1
  Delay2/1 -> data_out/1
  Detect Rise Positive/1 -> Sample Control Bus Creator/1

== system rx2/process divide/transport_block4/Subsystem3/ctrl_gen ==
  data_in : Inport
  valid_in : Inport  Port=2
  Delay : Delay  DelayLength=1  InitialCondition=0
  Delay1 : Delay  DelayLength=1  InitialCondition=0
  Delay2 : Delay  DelayLength=1  InitialCondition=0
  Detect Fall Nonpositive : hdlsllib/Logic and Bit Operations/Detect Fall Nonpositive  vinit=0  OutDataTypeStr=boolean
  Detect Rise Positive : hdlsllib/Logic and Bit Operations/Detect Rise Positive  vinit=0  OutDataTypeStr=boolean
  Sample Control Bus Creator : whdlutilities/Sample Control Bus Creator
  data_out : Outport
  ctrl_out : Outport  Port=2
  wires:
  Detect Rise Positive/1 -> Sample Control Bus Creator/1
  Delay2/1 -> data_out/1
  data_in/1 -> Delay2/1
  Delay1/1 -> Detect Rise Positive/1
  Delay/1 -> Sample Control Bus Creator/3
  Sample Control Bus Creator/1 -> ctrl_out/1
  valid_in/1 -> Delay1/1, Detect Fall Nonpositive/1, Delay/1
  Detect Fall Nonpositive/1 -> Sample Control Bus Creator/2

== system rx2/process divide/transport_block4/Subsystem4/ctrl_gen ==
  data_in : Inport
  valid_in : Inport  Port=2
  Delay : Delay  DelayLength=1  InitialCondition=0
  Delay1 : Delay  DelayLength=1  InitialCondition=0
  Delay2 : Delay  DelayLength=1  InitialCondition=0
  Detect Fall Nonpositive : hdlsllib/Logic and Bit Operations/Detect Fall Nonpositive  vinit=0  OutDataTypeStr=boolean
  Detect Rise Positive : hdlsllib/Logic and Bit Operations/Detect Rise Positive  vinit=0  OutDataTypeStr=boolean
  Sample Control Bus Creator : whdlutilities/Sample Control Bus Creator
  data_out : Outport
  ctrl_out : Outport  Port=2
  wires:
  Detect Fall Nonpositive/1 -> Sample Control Bus Creator/2
  valid_in/1 -> Delay/1, Detect Fall Nonpositive/1, Delay1/1
  Sample Control Bus Creator/1 -> ctrl_out/1
  Delay/1 -> Sample Control Bus Creator/3
  Delay1/1 -> Detect Rise Positive/1
  data_in/1 -> Delay2/1
  Delay2/1 -> data_out/1
  Detect Rise Positive/1 -> Sample Control Bus Creator/1

== system rx2/process divide/transport_block4/Subsystem5/ctrl_gen ==
  data_in : Inport
  valid_in : Inport  Port=2
  Delay : Delay  DelayLength=1  InitialCondition=0
  Delay1 : Delay  DelayLength=1  InitialCondition=0
  Delay2 : Delay  DelayLength=1  InitialCondition=0
  Detect Fall Nonpositive : hdlsllib/Logic and Bit Operations/Detect Fall Nonpositive  vinit=0  OutDataTypeStr=boolean
  Detect Rise Positive : hdlsllib/Logic and Bit Operations/Detect Rise Positive  vinit=0  OutDataTypeStr=boolean
  Sample Control Bus Creator : whdlutilities/Sample Control Bus Creator
  data_out : Outport
  ctrl_out : Outport  Port=2
  wires:
  Detect Fall Nonpositive/1 -> Sample Control Bus Creator/2
  valid_in/1 -> Delay/1, Detect Fall Nonpositive/1, Delay1/1
  Sample Control Bus Creator/1 -> ctrl_out/1
  Delay/1 -> Sample Control Bus Creator/3
  Delay1/1 -> Detect Rise Positive/1
  data_in/1 -> Delay2/1
  Delay2/1 -> data_out/1
  Detect Rise Positive/1 -> Sample Control Bus Creator/1

== system rx2/process divide/transport_block4/Subsystem6/ctrl_gen ==
  data_in : Inport
  valid_in : Inport  Port=2
  Delay : Delay  DelayLength=1  InitialCondition=0
  Delay1 : Delay  DelayLength=1  InitialCondition=0
  Delay2 : Delay  DelayLength=1  InitialCondition=0
  Detect Fall Nonpositive : hdlsllib/Logic and Bit Operations/Detect Fall Nonpositive  vinit=0  OutDataTypeStr=boolean
  Detect Rise Positive : hdlsllib/Logic and Bit Operations/Detect Rise Positive  vinit=0  OutDataTypeStr=boolean
  Sample Control Bus Creator : whdlutilities/Sample Control Bus Creator
  data_out : Outport
  ctrl_out : Outport  Port=2
  wires:
  Detect Fall Nonpositive/1 -> Sample Control Bus Creator/2
  valid_in/1 -> Delay/1, Detect Fall Nonpositive/1, Delay1/1
  Sample Control Bus Creator/1 -> ctrl_out/1
  Delay/1 -> Sample Control Bus Creator/3
  Delay1/1 -> Detect Rise Positive/1
  data_in/1 -> Delay2/1
  Delay2/1 -> data_out/1
  Detect Rise Positive/1 -> Sample Control Bus Creator/1

== system rx2/process divide/transport_block4/Subsystem7/ctrl_gen ==
  data_in : Inport
  valid_in : Inport  Port=2
  Delay : Delay  DelayLength=1  InitialCondition=0
  Delay1 : Delay  DelayLength=1  InitialCondition=0
  Delay2 : Delay  DelayLength=1  InitialCondition=0
  Detect Fall Nonpositive : hdlsllib/Logic and Bit Operations/Detect Fall Nonpositive  vinit=0  OutDataTypeStr=boolean
  Detect Rise Positive : hdlsllib/Logic and Bit Operations/Detect Rise Positive  vinit=0  OutDataTypeStr=boolean
  Sample Control Bus Creator : whdlutilities/Sample Control Bus Creator
  data_out : Outport
  ctrl_out : Outport  Port=2
  wires:
  Detect Fall Nonpositive/1 -> Sample Control Bus Creator/2
  valid_in/1 -> Delay/1, Detect Fall Nonpositive/1, Delay1/1
  Sample Control Bus Creator/1 -> ctrl_out/1
  Delay/1 -> Sample Control Bus Creator/3
  Delay1/1 -> Detect Rise Positive/1
  data_in/1 -> Delay2/1
  Delay2/1 -> data_out/1
  Detect Rise Positive/1 -> Sample Control Bus Creator/1

== system rx2/process divide/transport_block4/Subsystem8/ctrl_gen ==
  data_in : Inport
  valid_in : Inport  Port=2
  Delay : Delay  DelayLength=1  InitialCondition=0
  Delay1 : Delay  DelayLength=1  InitialCondition=0
  Delay2 : Delay  DelayLength=1  InitialCondition=0
  Detect Fall Nonpositive : hdlsllib/Logic and Bit Operations/Detect Fall Nonpositive  vinit=0  OutDataTypeStr=boolean
  Detect Rise Positive : hdlsllib/Logic and Bit Operations/Detect Rise Positive  vinit=0  OutDataTypeStr=boolean
  Sample Control Bus Creator : whdlutilities/Sample Control Bus Creator
  data_out : Outport
  ctrl_out : Outport  Port=2
  wires:
  Detect Fall Nonpositive/1 -> Sample Control Bus Creator/2
  valid_in/1 -> Delay/1, Detect Fall Nonpositive/1, Delay1/1
  Sample Control Bus Creator/1 -> ctrl_out/1
  Delay/1 -> Sample Control Bus Creator/3
  Delay1/1 -> Detect Rise Positive/1
  data_in/1 -> Delay2/1
  Delay2/1 -> data_out/1
  Detect Rise Positive/1 -> Sample Control Bus Creator/1

== system rx2/process divide/transport_block4/Subsystem9/ctrl_gen ==
  data_in : Inport
  valid_in : Inport  Port=2
  Delay : Delay  DelayLength=1  InitialCondition=0
  Delay1 : Delay  DelayLength=1  InitialCondition=0
  Delay2 : Delay  DelayLength=1  InitialCondition=0
  Detect Fall Nonpositive : hdlsllib/Logic and Bit Operations/Detect Fall Nonpositive  vinit=0  OutDataTypeStr=boolean
  Detect Rise Positive : hdlsllib/Logic and Bit Operations/Detect Rise Positive  vinit=0  OutDataTypeStr=boolean
  Sample Control Bus Creator : whdlutilities/Sample Control Bus Creator
  data_out : Outport
  ctrl_out : Outport  Port=2
  wires:
  Detect Fall Nonpositive/1 -> Sample Control Bus Creator/2
  valid_in/1 -> Delay/1, Detect Fall Nonpositive/1, Delay1/1
  Sample Control Bus Creator/1 -> ctrl_out/1
  Delay/1 -> Sample Control Bus Creator/3
  Delay1/1 -> Detect Rise Positive/1
  data_in/1 -> Delay2/1
  Delay2/1 -> data_out/1
  Detect Rise Positive/1 -> Sample Control Bus Creator/1
